simulink model "Horizon_Array_Calculation"  (R2016b)
settings: Solver=FixedStepDiscrete  StartTime=0.0  StopTime=inf  FixedStep=HrznAryCalcn.tiSimnTiStep_C  RelTol=1e-3  EnableMultiTasking=on
settings Model: Creator=djuenema  LastModifiedBy=djuenema
settings DataIOCC: SaveFormat=StructureWithTime  SaveOutput=off  DSMLogging=off  VisualizeSimOutput=off  SaveTime=off  SignalLoggingName=Results
settings OptimizationCC: BlockReduction=off  ConditionallyExecuteInputs=off  LifeSpan=inf
settings DebuggingCC: AllowSymbolicDim=off  SFUnexpectedBacktrackingDiag=warning  SFNoUnconditionalDefaultTransitionDiag=warning  SFExecutionAtInitializationDiag=none
settings ModelReferenceCC: ModelReferenceNumInstancesAllowed=Single  PropagateSignalLabelsOutOfModel=off
settings GRTTargetCC: TargetLangStandard=C89/C90 (ANSI)
settings ConfigComp: CovMetricSettings=dw  CovHtmlReporting=on  CovSaveCumulativeToWorkspaceVar=on  CovSaveSingleToWorkspaceVar=on  CovExternalEMLEnable=off

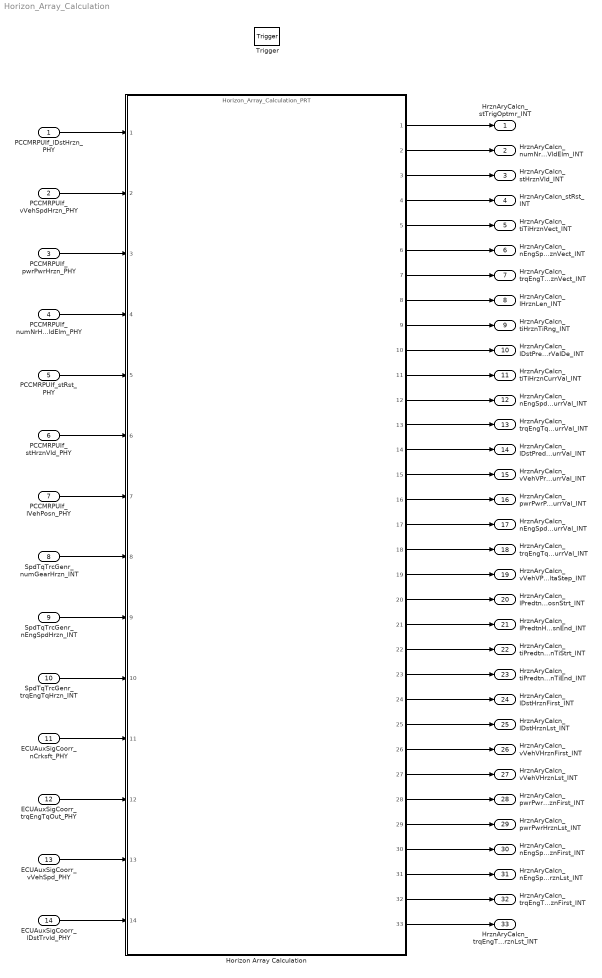
== system Horizon_Array_Calculation ==
  PCCMRPUIf_lDstHrzn_PHY : Inport
  PCCMRPUIf_vVehSpdHrzn_PHY : Inport  Port=2
  PCCMRPUIf_pwrPwrHrzn_PHY : Inport  Port=3
  PCCMRPUIf_numNrHrznVldElm_PHY : Inport  Port=4
  PCCMRPUIf_stRst_PHY : Inport  Port=5
  PCCMRPUIf_stHrznVld_PHY : Inport  Port=6
  PCCMRPUIf_lVehPosn_PHY : Inport  Port=7
  SpdTqTrcGenr_numGearHrzn_INT : Inport  Port=8
  SpdTqTrcGenr_nEngSpdHrzn_INT : Inport  Port=9
  SpdTqTrcGenr_trqEngTqHrzn_INT : Inport  Port=10
  ECUAuxSigCoorr_nCrksft_PHY : Inport  Port=11
  ECUAuxSigCoorr_trqEngTqOut_PHY : Inport  Port=12
  ECUAuxSigCoorr_vVehSpd_PHY : Inport  Port=13
  ECUAuxSigCoorr_lDstTrvld_PHY : Inport  Port=14
  Trigger : TriggerPort  TriggerType=function-call  VariantControl=Variant  PortDimensions=1
  Horizon Array Calculation : ModelReference  ModelNameDialog=Horizon_Array_Calculation_PRT.slxp  ModelReferenceVersion=1.3  CopyOfModelProtected=on
  HrznAryCalcn_stTrigOptmr_INT : Outport
  HrznAryCalcn_numNrHrznVldElm_INT : Outport  Port=2
  HrznAryCalcn_stHrznVld_INT : Outport  Port=3
  HrznAryCalcn_stRst_INT : Outport  Port=4
  HrznAryCalcn_tiTiHrznVect_INT : Outport  Port=5
  HrznAryCalcn_nEngSpdHrznVect_INT : Outport  Port=6
  HrznAryCalcn_trqEngTqHrznVect_INT : Outport  Port=7
  HrznAryCalcn_lHrznLen_INT : Outport  Port=8
  HrznAryCalcn_tiHrznTiRng_INT : Outport  Port=9
  HrznAryCalcn_lDstPredCurrValDe_INT : Outport  Port=10
  HrznAryCalcn_tiTiHrznCurrVal_INT : Outport  Port=11
  HrznAryCalcn_nEngSpdHrznCurrVal_INT : Outport  Port=12
  HrznAryCalcn_trqEngTqHrznCurrVal_INT : Outport  Port=13
  HrznAryCalcn_lDstPredCurrVal_INT : Outport  Port=14
  HrznAryCalcn_vVehVPredCurrVal_INT : Outport  Port=15
  HrznAryCalcn_pwrPwrPredCurrVal_INT : Outport  Port=16
  HrznAryCalcn_nEngSpdPredTrcCurrVal_INT : Outport  Port=17
  HrznAryCalcn_trqEngTqPredTrcCurrVal_INT : Outport  Port=18
  HrznAryCalcn_vVehVPredDeltaStep_INT : Outport  Port=19
  HrznAryCalcn_lPredtnHrznPosnStrt_INT : Outport  Port=20
  HrznAryCalcn_lPredtnHrznPosnEnd_INT : Outport  Port=21
  HrznAryCalcn_tiPredtnHrznTiStrt_INT : Outport  Port=22
  HrznAryCalcn_tiPredtnHrznTiEnd_INT : Outport  Port=23
  HrznAryCalcn_lDstHrznFirst_INT : Outport  Port=24
  HrznAryCalcn_lDstHrznLst_INT : Outport  Port=25
  HrznAryCalcn_vVehVHrznFirst_INT : Outport  Port=26
  HrznAryCalcn_vVehVHrznLst_INT : Outport  Port=27
  HrznAryCalcn_pwrPwrHrznFirst_INT : Outport  Port=28
  HrznAryCalcn_pwrPwrHrznLst_INT : Outport  Port=29
  HrznAryCalcn_nEngSpdHrznFirst_INT : Outport  Port=30
  HrznAryCalcn_nEngSpdHrznLst_INT : Outport  Port=31
  HrznAryCalcn_trqEngTqHrznFirst_INT : Outport  Port=32
  HrznAryCalcn_trqEngTqHrznLst_INT : Outport  Port=33
  wires:
  SpdTqTrcGenr_trqEngTqHrzn_INT/1 -> Horizon Array Calculation/10
  PCCMRPUIf_lDstHrzn_PHY/1 -> Horizon Array Calculation/1
  PCCMRPUIf_pwrPwrHrzn_PHY/1 -> Horizon Array Calculation/3
  PCCMRPUIf_numNrHrznVldElm_PHY/1 -> Horizon Array Calculation/4
  SpdTqTrcGenr_nEngSpdHrzn_INT/1 -> Horizon Array Calculation/9
  PCCMRPUIf_lVehPosn_PHY/1 -> Horizon Array Calculation/7
  PCCMRPUIf_vVehSpdHrzn_PHY/1 -> Horizon Array Calculation/2
  SpdTqTrcGenr_numGearHrzn_INT/1 -> Horizon Array Calculation/8
  PCCMRPUIf_stHrznVld_PHY/1 -> Horizon Array Calculation/6
  PCCMRPUIf_stRst_PHY/1 -> Horizon Array Calculation/5
  Horizon Array Calculation/4 -> HrznAryCalcn_stRst_INT/1
  Horizon Array Calculation/1 -> HrznAryCalcn_stTrigOptmr_INT/1
  Horizon Array Calculation/6 -> HrznAryCalcn_nEngSpdHrznVect_INT/1
  Horizon Array Calculation/5 -> HrznAryCalcn_tiTiHrznVect_INT/1
  Horizon Array Calculation/3 -> HrznAryCalcn_stHrznVld_INT/1
  Horizon Array Calculation/2 -> HrznAryCalcn_numNrHrznVldElm_INT/1
  Horizon Array Calculation/17 -> HrznAryCalcn_nEngSpdPredTrcCurrVal_INT/1
  Horizon Array Calculation/15 -> HrznAryCalcn_vVehVPredCurrVal_INT/1
  Horizon Array Calculation/7 -> HrznAryCalcn_trqEngTqHrznVect_INT/1
  Horizon Array Calculation/13 -> HrznAryCalcn_trqEngTqHrznCurrVal_INT/1
  Horizon Array Calculation/16 -> HrznAryCalcn_pwrPwrPredCurrVal_INT/1
  Horizon Array Calculation/18 -> HrznAryCalcn_trqEngTqPredTrcCurrVal_INT/1
  Horizon Array Calculation/8 -> HrznAryCalcn_lHrznLen_INT/1
  Horizon Array Calculation/11 -> HrznAryCalcn_tiTiHrznCurrVal_INT/1
  Horizon Array Calculation/9 -> HrznAryCalcn_tiHrznTiRng_INT/1
  Horizon Array Calculation/14 -> HrznAryCalcn_lDstPredCurrVal_INT/1
  Horizon Array Calculation/10 -> HrznAryCalcn_lDstPredCurrValDe_INT/1
  Horizon Array Calculation/12 -> HrznAryCalcn_nEngSpdHrznCurrVal_INT/1
  ECUAuxSigCoorr_nCrksft_PHY/1 -> Horizon Array Calculation/11
  ECUAuxSigCoorr_trqEngTqOut_PHY/1 -> Horizon Array Calculation/12
  Horizon Array Calculation/19 -> HrznAryCalcn_vVehVPredDeltaStep_INT/1
  Horizon Array Calculation/20 -> HrznAryCalcn_lPredtnHrznPosnStrt_INT/1
  Horizon Array Calculation/21 -> HrznAryCalcn_lPredtnHrznPosnEnd_INT/1
  Horizon Array Calculation/22 -> HrznAryCalcn_tiPredtnHrznTiStrt_INT/1
  Horizon Array Calculation/23 -> HrznAryCalcn_tiPredtnHrznTiEnd_INT/1
  ECUAuxSigCoorr_vVehSpd_PHY/1 -> Horizon Array Calculation/13
  ECUAuxSigCoorr_lDstTrvld_PHY/1 -> Horizon Array Calculation/14
  Horizon Array Calculation/24 -> HrznAryCalcn_lDstHrznFirst_INT/1
  Horizon Array Calculation/29 -> HrznAryCalcn_pwrPwrHrznLst_INT/1
  Horizon Array Calculation/27 -> HrznAryCalcn_vVehVHrznLst_INT/1
  Horizon Array Calculation/26 -> HrznAryCalcn_vVehVHrznFirst_INT/1
  Horizon Array Calculation/28 -> HrznAryCalcn_pwrPwrHrznFirst_INT/1
  Horizon Array Calculation/25 -> HrznAryCalcn_lDstHrznLst_INT/1
  Horizon Array Calculation/30 -> HrznAryCalcn_nEngSpdHrznFirst_INT/1
  Horizon Array Calculation/31 -> HrznAryCalcn_nEngSpdHrznLst_INT/1
  Horizon Array Calculation/32 -> HrznAryCalcn_trqEngTqHrznFirst_INT/1
  Horizon Array Calculation/33 -> HrznAryCalcn_trqEngTqHrznLst_INT/1
